simulink model "thermal_decay"  (R2026a)
settings: Solver=VariableStepAuto  StopTime=50

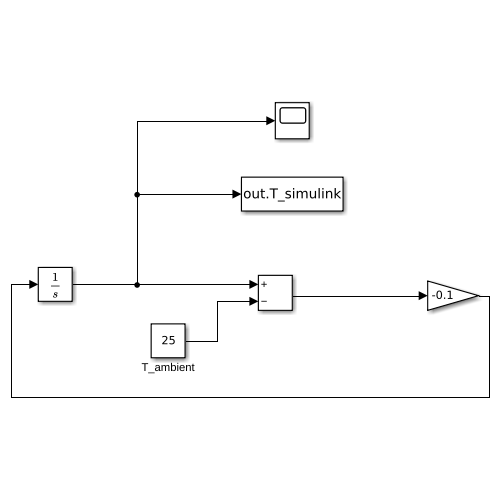
[thumbnail: Simulink's stored preview of the top-level diagram]
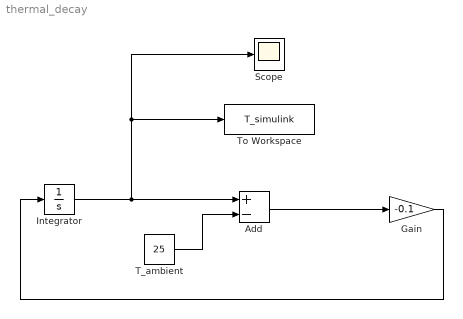
== system thermal_decay ==
  Add : Sum  Inputs=+-
  Gain : Gain  Gain=-0.1
  Integrator : Integrator  InitialCondition=100
  Scope : Scope
      settings: ActiveDisplayYMinimum=16.19351428738992  ActiveDisplayYMaximum=109.31183174584557
  T_ambient : Constant  Value=25
  To Workspace : ToWorkspace  VariableName=T_simulink  SaveFormat=Timeseries  SampleTime=-1
  wires:
  Integrator/1 -> To Workspace/1, Scope/1, Add/1
  T_ambient/1 -> Add/2
  Add/1 -> Gain/1
  Gain/1 -> Integrator/1
